simulink model "MSDR_v1.1"  (R2018a)
settings: Solver=ode3  StartTime=0.0  StopTime=21600  FixedStep=0.05
values from neighbouring files (symbols this model uses):
  a_f = -3.22E-5    (= -3.22e-05)    [MSDR_parameters.m]
  a_g = +2.35E-5    (= 2.35e-05)    [MSDR_parameters.m]
  A_s = 1.2245    [MSDR_parameters.m]
  beta = [0.000223, 0.001457, 0.001307, 0.002628, 0.000766, 0.000280]    [MSDR_parameters.m]
  beta_t = sum(beta)    [MSDR_parameters.m]
  ce1 = 1.2471e-07    [MSDR_parameters.m]
  ce2 = 5.3816e-14    [MSDR_parameters.m]
  ce3 = 3.3721e-08    [MSDR_parameters.m]
  Cp_fw = 3200.448e-6    (= 0.003200448)    [MSDR_parameters.m]
  Cp_hr = 0.0021520    (= 0.002152)    [MSDR_parameters.m]
  Cp_p = Cp_s_shx    (= 0.00154912)    [MSDR_parameters.m]
  Cp_s = Cp_s*1e-6    (= 3.588208e-09)    [MSDR_parameters.m]
  Cp_s_shx = 1549.12e-6    (= 0.00154912)    [MSDR_parameters.m]
  Cp_sc = 4761.392e-6    (= 0.004761392)    [MSDR_parameters.m]
  Cp_w = 456.056e-6    (= 0.000456056)    [MSDR_parameters.m]
  D_it = 0.0141478    [MSDR_parameters.m]
  D_ot = 0.015875    [MSDR_parameters.m]
  dHs_dPs = -0.042433622114357    (= -0.0424336221144)    [MSDR_parameters.m]
  eta_hp_isen = 0.861    [MSDR_parameters.m]
  eta_lp_isen = 0.861    [MSDR_parameters.m]
  gamma_I = 5.1135e-2    (= 0.051135)    [MSDR_parameters.m]
  gamma_Xe = 1.1628e-2    (= 0.011628)    [MSDR_parameters.m]
  H_fwh1 = 0.46009    [MSDR_parameters.m]
  h_fwh1 = 0.5927    [MSDR_parameters.m]
  H_fwh2 = 0.6784    [MSDR_parameters.m]
  h_fwh2 = 0.5927    [MSDR_parameters.m]
  H_lp_isen = 958.4*1054.35e-6/0.45359237    (= 2.22774699671)    [MSDR_parameters.m]
  H_nc = 3.2952    [MSDR_parameters.m]
  h_pw = h_s_shx    (= 0.00567446)    [MSDR_parameters.m]
  H_rh = 2.8115    [MSDR_parameters.m]
  h_wb = 13349.334646671E-6    (= 0.0133493346467)    [MSDR_parameters.m]
  h_ws = 5732.378387768E-6    (= 0.00573237838777)    [MSDR_parameters.m]
  h_wsc = 8385.005556375E-6    (= 0.00838500555638)    [MSDR_parameters.m]
  hA_fg = [h_fg*A_fg/2, h_fg*A_fg/2]    [MSDR_parameters.m]
  hA_p_phx1 = h_p_phx*A_p_phx    [MSDR_parameters.m]
  hA_p_phx2 = h_p_phx*A_p_phx    [MSDR_parameters.m]
  hA_p_phx3 = h_p_phx*A_p_phx    [MSDR_parameters.m]
  hA_p_phx4 = h_p_phx*A_p_phx    [MSDR_parameters.m]
  hA_p_phx5 = h_p_phx*A_p_phx    [MSDR_parameters.m]
  hA_p_phx6 = h_p_phx*A_p_phx    [MSDR_parameters.m]
  hA_p_shx1 = h_p_shx*A_p_shx    [MSDR_parameters.m]
  hA_p_shx2 = h_p_shx*A_p_shx    [MSDR_parameters.m]
  hA_p_shx3 = h_p_shx*A_p_shx    [MSDR_parameters.m]
  hA_p_shx4 = h_p_shx*A_p_shx    [MSDR_parameters.m]
  hA_p_shx5 = h_p_shx*A_p_shx    [MSDR_parameters.m]
  hA_p_shx6 = h_p_shx*A_p_shx    [MSDR_parameters.m]
  hA_s_phx1 = h_s_phx*A_s_phx    [MSDR_parameters.m]
  hA_s_phx2 = h_s_phx*A_s_phx    [MSDR_parameters.m]
  hA_s_phx3 = h_s_phx*A_s_phx    [MSDR_parameters.m]
  hA_s_phx4 = h_s_phx*A_s_phx    [MSDR_parameters.m]
  hA_s_phx5 = h_s_phx*A_s_phx    [MSDR_parameters.m]
  hA_s_phx6 = h_s_phx*A_s_phx    [MSDR_parameters.m]
  hA_s_shx1 = h_s_shx*A_s_shx    [MSDR_parameters.m]
  hA_s_shx2 = h_s_shx*A_s_shx    [MSDR_parameters.m]
  hA_s_shx3 = h_s_shx*A_s_shx    [MSDR_parameters.m]
  hA_s_shx4 = h_s_shx*A_s_shx    [MSDR_parameters.m]
  hA_s_shx5 = h_s_shx*A_s_shx    [MSDR_parameters.m]
  hA_s_shx6 = h_s_shx*A_s_shx    [MSDR_parameters.m]
  I_0 = gamma_I*Sig_f_msdr*phi_0/lam_I    (= 4.38204721773e+16)    [MSDR_parameters.m]
  Ifa = [0.25, 0.25]    [MSDR_parameters.m]
  Ifb = [0.25, 0.25]    [MSDR_parameters.m]
  Ig = [0.5, 0.5]    [MSDR_parameters.m]
  K_1 = 11.632248097704855    (= 11.6322480977)    [MSDR_parameters.m]
  K_4 = b(1)    [MSDR_parameters.m]
  K_5 = a(1)    [MSDR_parameters.m]
  K_b = 12.834854076292217    (= 12.8348540763)    [MSDR_parameters.m]
  K_b_hp = 0.1634    [MSDR_parameters.m]
  K_b_lp = 0.2174    [MSDR_parameters.m]
  K_sc = -17.615718797133468    (= -17.6157187971)    [MSDR_parameters.m]
  ka = [0.235, 0.235]    [MSDR_parameters.m]
  kb = [0.235, 0.235]    [MSDR_parameters.m]
  kga = [0.015, 0.015]    [MSDR_parameters.m]
  kgb = [0.015, 0.015]    [MSDR_parameters.m]
  L = 8.5344    [MSDR_parameters.m]
  L_b = 2.3645    [MSDR_parameters.m]
  L_s = 4.723    [MSDR_parameters.m]
  Lam = 2.400E-04    (= 0.00024)    [MSDR_parameters.m]
  lam = [0.0124, 0.0305, 0.111, 0.301, 1.14, 3.01]    [MSDR_parameters.m]
  lam_bubl = 2.0e-2    (= 0.02)    [MSDR_parameters.m]
  lam_I = 2.875e-5    (= 2.875e-05)    [MSDR_parameters.m]
  lam_Xe = 2.0916e-5    (= 2.0916e-05)    [MSDR_parameters.m]
  m_3m = W_3*2    (= 8618.207327)    [MSDR_parameters.m]
  m_fm = W_f*2    (= 9978.96)    [MSDR_parameters.m]
  m_sb = 1717    [MSDR_parameters.m]
  M_stm = 0.018    [MSDR_parameters.m]
  mb_cpb = 2.689619410657651e+00    (= 2.68961941066)    [MSDR_parameters.m]
  mcp_fa = mfa*Cp_f    [MSDR_parameters.m]
  mcp_fb = mfb*Cp_f    [MSDR_parameters.m]
  mcp_g = mg*Cp_g    [MSDR_parameters.m]
  mcp_p_phx1 = Cp_p_phx*mp_phx1    [MSDR_parameters.m]
  mcp_p_phx2 = Cp_p_phx*mp_phx2    [MSDR_parameters.m]
  mcp_p_phx3 = Cp_p_phx*mp_phx3    [MSDR_parameters.m]
  mcp_p_phx4 = Cp_p_phx*mp_phx4    [MSDR_parameters.m]
  mcp_p_phx5 = Cp_p_phx*mp_phx5    [MSDR_parameters.m]
  mcp_p_phx6 = Cp_p_phx*mp_phx6    [MSDR_parameters.m]
  mcp_p_shx1 = Cp_p_shx*mp_shx1    [MSDR_parameters.m]
  mcp_p_shx2 = Cp_p_shx*mp_shx2    [MSDR_parameters.m]
  mcp_p_shx3 = Cp_p_shx*mp_shx3    [MSDR_parameters.m]
  mcp_p_shx4 = Cp_p_shx*mp_shx4    [MSDR_parameters.m]
  mcp_p_shx5 = Cp_p_shx*mp_shx5    [MSDR_parameters.m]
  mcp_p_shx6 = Cp_p_shx*mp_shx6    [MSDR_parameters.m]
  mcp_s_phx1 = Cp_s_phx*ms_phx1    [MSDR_parameters.m]
  mcp_s_phx2 = Cp_s_phx*ms_phx2    [MSDR_parameters.m]
  mcp_s_phx3 = Cp_s_phx*ms_phx3    [MSDR_parameters.m]
  mcp_s_phx4 = Cp_s_phx*ms_phx4    [MSDR_parameters.m]
  mcp_s_phx5 = Cp_s_phx*ms_phx5    [MSDR_parameters.m]
  mcp_s_phx6 = Cp_s_phx*ms_phx6    [MSDR_parameters.m]
  mcp_s_shx1 = Cp_s_shx*ms_shx1    [MSDR_parameters.m]
  mcp_s_shx2 = Cp_s_shx*ms_shx1    [MSDR_parameters.m]
  mcp_s_shx3 = Cp_s_shx*ms_shx1    [MSDR_parameters.m]
  mcp_s_shx4 = Cp_s_shx*ms_shx1    [MSDR_parameters.m]
  mcp_s_shx5 = Cp_s_shx*ms_shx1    [MSDR_parameters.m]
  mcp_s_shx6 = Cp_s_shx*ms_shx1    [MSDR_parameters.m]
  mcp_t_phx1 = Cp_t_phx*mt_phx1    [MSDR_parameters.m]
  mcp_t_phx2 = Cp_t_phx*mt_phx2    [MSDR_parameters.m]
  mcp_t_phx3 = Cp_t_phx*mt_phx3    [MSDR_parameters.m]
  mcp_t_phx4 = Cp_t_phx*mt_phx4    [MSDR_parameters.m]
  mcp_t_phx5 = Cp_t_phx*mt_phx5    [MSDR_parameters.m]
  mcp_t_phx6 = Cp_t_phx*mt_phx6    [MSDR_parameters.m]
  mcp_t_shx1 = Cp_t_phx*mt_shx1    [MSDR_parameters.m]
  ... (+177 more)
undefined symbols (not defined in the file or in its folder): C0, H_rh_table, H_rh_table1, H_rh_table2, H_rhvap_table, H_s_table, H_table, hA_p_thx1, hA_p_thx2, hA_p_thx3, hA_s_thx1, hA_s_thx2, hA_s_thx3, mcp_p_thx1, mcp_p_thx2, mcp_p_thx3, mcp_s_thx1, mcp_s_thx2, mcp_s_thx3, mcp_t_thx1, mcp_t_thx2, mcp_t_thx3, mp_thx1, mp_thx2, mp_thx3, ms_thx1, ms_thx2, ms_thx3, P_nc_table, P_rh_table, P_rh_table1, pres_table, rho_rh_table, rho_table, SV_nc_table, T0_p_thx1, T0_p_thx2, T0_p_thx3, T0_s_thx1, T0_s_thx2, T0_s_thx3, T0_t_thx1, T0_t_thx2, T0_t_thx3, temp_table, u14, Wp_thx1, Wp_thx2
libraries: simulink x13
(part 1 of 6)
settings Model: Creator=viikr  LastModifiedBy=Vikram Singh
settings SolverCC: AlgebraicLoopSolver=LineSearch

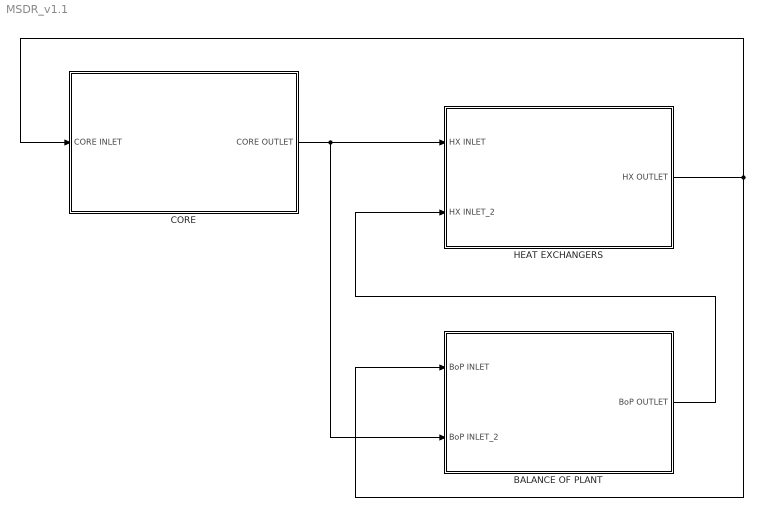
== system MSDR_v1.1 ==
  BALANCE OF PLANT : Subsystem
  CORE : Subsystem
  HEAT EXCHANGERS : Subsystem
  wires:
  BALANCE OF PLANT/1(BoP OUTLET) -> HEAT EXCHANGERS/2(HX INLET_2)
  HEAT EXCHANGERS/1(HX OUTLET) -> BALANCE OF PLANT/1(BoP INLET), CORE/1(CORE INLET)
  CORE/1(CORE OUTLET) -> BALANCE OF PLANT/2(BoP INLET_2), HEAT EXCHANGERS/1(HX INLET)

== system MSDR_v1.1/BALANCE OF PLANT ==
  In Bus Element : Inport  PortName=BoP INLET  Element=HX HITEC OUTLET TEMPERATURE
  In Bus Element1 : Inport  Port=2  PortName=BoP INLET_2  Element=CORE POWER
  Constant : Constant  Value=425
  POWER : Subsystem
  Bus Element Out2 : Outport  PortName=BoP OUTLET  Element=BoP HITEC OUTLET TEMPERATURE
  wires:
  In Bus Element/1 -> POWER/1(HITEC_INLET)
  In Bus Element1/1 -> POWER/2(POWER LEVEL)
  POWER/1(HITEC_OUTLET) -> Bus Element Out2/1

== system MSDR_v1.1/CORE ==
  In Bus Element2 : Inport  PortName=CORE INLET  Element=FUEL HEAT TRANSFER FRACTION
  In Bus Element : Inport  PortName=CORE INLET  Element=HX FUEL OUTLET TEMPERATURE
  In Bus Element1 : Inport  PortName=CORE INLET  Element=FUEL FLOW FRACTION
  CORE HEAT TRANSFER : Subsystem
  CORE TO HX DELAY : VariableTransportDelay  MaximumDelay=10000000  InitialOutput=T0_fb(2)
  PKE SOLVER : Subsystem
  REACTIVITY : Subsystem
  REACTIVITY1 : Subsystem
  Tf_out : Fcn  Expr=u[7]
  VAR DELAY FUNC : Fcn  Expr=tau_c_hx/u
  Bus Element Out2 : Outport  PortName=CORE OUTLET  Element=CORE FUEL OUTLET TEMPERATURE
  Bus Element Out1 : Outport  PortName=CORE OUTLET  Element=CORE POWER
  wires:
  Tf_out/1 -> CORE TO HX DELAY/1
  CORE HEAT TRANSFER/1(CORE TEMPERATURES) -> [Tf_out], Tf_out/1
  [Tf_out] -> REACTIVITY/1(CORE TEMPERATURES)
  PKE SOLVER/1(FRACTIONAL NEUTRON DENSITY) -> Bus Element Out1/1, [Frac_neut]
  [Frac_neut] -> CORE HEAT TRANSFER/1(FRACTIONAL NEUTRON DENSITY)
  REACTIVITY/1(TOTAL REACTIVITY FEEDBACK) -> [rho_tot]
  [flow_frac] -> PKE SOLVER/2(FLOW FRACTION)
  [flow_frac] -> CORE HEAT TRANSFER/3(FLOW FRACTION)
  [hA_frac] -> CORE HEAT TRANSFER/4(HEAT TRANSFER FRACTION)
  CORE TO HX DELAY/1 -> Bus Element Out2/1
  [flow_frac] -> VAR DELAY FUNC/1
  VAR DELAY FUNC/1 -> CORE TO HX DELAY/2
  [Tf_in] -> CORE HEAT TRANSFER/2(FUEL INLET TEMPERATURE)
  REACTIVITY1/1(drho_Xe) -> [drho_Xe]
  [Frac_neut] -> REACTIVITY1/1(n0)
  In Bus Element1/1 -> [flow_frac]
  In Bus Element2/1 -> [hA_frac]
  In Bus Element/1 -> [Tf_in]
  [drho_Xe] -> REACTIVITY/2(XENON REACTIVITY)
  [rho_tot] -> PKE SOLVER/1(REACTIVITY FEEDBACK)

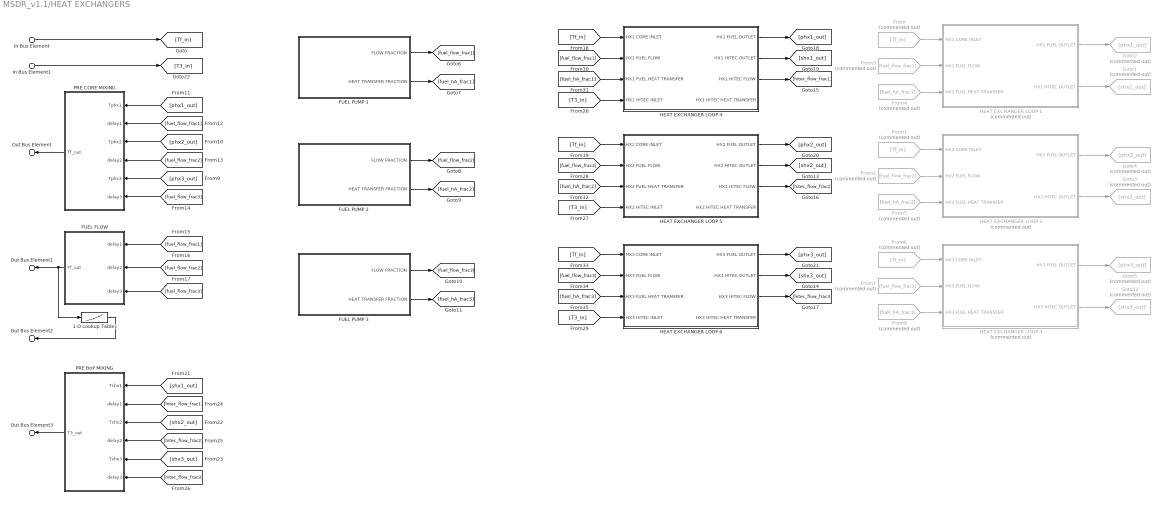
== system MSDR_v1.1/HEAT EXCHANGERS ==
  In Bus Element : Inport  PortName=HX INLET  Element=CORE FUEL OUTLET TEMPERATURE
  In Bus Element1 : Inport  Port=2  PortName=HX INLET_2  Element=BoP HITEC OUTLET TEMPERATURE
  1-D Lookup Table1 : Lookup_n-D  NumberOfTableDimensions=1  BreakpointsForDimension1=xdat  Table=ydat  InternalRulePriority=Speed  RndMeth=Simplest  InputSameDT=on
  FUEL FLOW : Subsystem
  FUEL PUMP 1 : Subsystem
  FUEL PUMP 2 : Subsystem
  FUEL PUMP 3 : Subsystem
  From : From  Commented=on  GotoTag=Tf_in
  From1 : From  Commented=on  GotoTag=Tf_in
  From2 : From  Commented=on  GotoTag=fuel_flow_frac2
  From3 : From  Commented=on  GotoTag=fuel_flow_frac1
  From4 : From  Commented=on  GotoTag=fuel_hA_frac1
  From5 : From  Commented=on  GotoTag=fuel_hA_frac2
  From6 : From  Commented=on  GotoTag=Tf_in
  From7 : From  Commented=on  GotoTag=fuel_flow_frac3
  From8 : From  Commented=on  GotoTag=fuel_hA_frac3
  Goto1 : Goto  Commented=on  GotoTag=shx1_out
  Goto12 : Goto  Commented=on  GotoTag=shx3_out
  Goto2 : Goto  Commented=on  GotoTag=phx1_out
  Goto3 : Goto  Commented=on  GotoTag=shx2_out
  Goto4 : Goto  Commented=on  GotoTag=phx2_out
  Goto5 : Goto  Commented=on  GotoTag=phx3_out
  HEAT EXCHANGER LOOP 1 : Subsystem  Commented=on
  HEAT EXCHANGER LOOP 2 : Subsystem  Commented=on
  HEAT EXCHANGER LOOP 3 : Subsystem  Commented=on
  HEAT EXCHANGER LOOP 4 : Subsystem
  HEAT EXCHANGER LOOP 5 : Subsystem
  HEAT EXCHANGER LOOP 6 : Subsystem
  PRE BoP MIXING : Subsystem
  PRE CORE MIXING : Subsystem
  Out Bus Element : Outport  PortName=HX OUTLET  Element=HX FUEL OUTLET TEMPERATURE
  Out Bus Element1 : Outport  PortName=HX OUTLET  Element=FUEL FLOW FRACTION
  Out Bus Element2 : Outport  PortName=HX OUTLET  Element=FUEL HEAT TRANSFER FRACTION
  Out Bus Element3 : Outport  PortName=HX OUTLET  Element=HX HITEC OUTLET TEMPERATURE
  wires:
  From/1 -> HEAT EXCHANGER LOOP 1/1(HX1 CORE INLET)
  From3/1 -> HEAT EXCHANGER LOOP 1/2(HX1 FUEL FLOW)
  From4/1 -> HEAT EXCHANGER LOOP 1/3(HX1 FUEL HEAT TRANSFER)
  From1/1 -> HEAT EXCHANGER LOOP 2/1(HX2 CORE INLET)
  From5/1 -> HEAT EXCHANGER LOOP 2/3(HX2 FUEL HEAT TRANSFER)
  From2/1 -> HEAT EXCHANGER LOOP 2/2(HX2 FUEL FLOW)
  From6/1 -> HEAT EXCHANGER LOOP 3/1(HX3 CORE INLET)
  From7/1 -> HEAT EXCHANGER LOOP 3/2(HX3 FUEL FLOW)
  From8/1 -> HEAT EXCHANGER LOOP 3/3(HX3 FUEL HEAT TRANSFER)
  In Bus Element/1 -> [Tf_in]
  HEAT EXCHANGER LOOP 1/1(HX1 FUEL OUTLET) -> Goto2/1
  HEAT EXCHANGER LOOP 2/1(HX2 FUEL OUTLET) -> Goto4/1
  HEAT EXCHANGER LOOP 3/1(HX3 FUEL OUTLET) -> Goto5/1
  FUEL PUMP 1/1(FLOW FRACTION) -> [fuel_flow_frac1]
  FUEL PUMP 1/2(HEAT TRANSFER FRACTION) -> [fuel_hA_frac1]
  FUEL PUMP 2/2(HEAT TRANSFER FRACTION) -> [fuel_hA_frac2]
  FUEL PUMP 2/1(FLOW FRACTION) -> [fuel_flow_frac2]
  FUEL PUMP 3/2(HEAT TRANSFER FRACTION) -> [fuel_hA_frac3]
  FUEL PUMP 3/1(FLOW FRACTION) -> [fuel_flow_frac3]
  [phx1_out] -> PRE CORE MIXING/1(Tphx1)
  [fuel_flow_frac1] -> PRE CORE MIXING/2(delay1)
  [phx2_out] -> PRE CORE MIXING/3(Tphx2)
  [fuel_flow_frac2] -> PRE CORE MIXING/4(delay2)
  [phx3_out] -> PRE CORE MIXING/5(Tphx3)
  [fuel_flow_frac3] -> PRE CORE MIXING/6(delay3)
  PRE CORE MIXING/1(Tf_out) -> Out Bus Element/1
  [fuel_flow_frac2] -> FUEL FLOW/2(delay2)
  [fuel_flow_frac1] -> FUEL FLOW/1(delay1)
  [fuel_flow_frac3] -> FUEL FLOW/3(delay3)
  FUEL FLOW/1(Tf_out) -> 1-D Lookup Table1/1, Out Bus Element1/1
  1-D Lookup Table1/1 -> Out Bus Element2/1
  [hitec_flow_frac2] -> PRE BoP MIXING/4(delay2)
  [hitec_flow_frac1] -> PRE BoP MIXING/2(delay1)
  [shx2_out] -> PRE BoP MIXING/3(Tshx2)
  [shx3_out] -> PRE BoP MIXING/5(Tshx3)
  [hitec_flow_frac3] -> PRE BoP MIXING/6(delay3)
  [shx1_out] -> PRE BoP MIXING/1(Tshx1)
  PRE BoP MIXING/1(T3_out) -> Out Bus Element3/1
  HEAT EXCHANGER LOOP 1/2(HX1 HITEC OUTLET) -> Goto1/1
  HEAT EXCHANGER LOOP 2/2(HX2 HITEC OUTLET) -> Goto3/1
  HEAT EXCHANGER LOOP 3/2(HX3 HITEC OUTLET) -> Goto12/1
  HEAT EXCHANGER LOOP 5/2(HX2 HITEC OUTLET) -> [shx2_out]
  [T3_in] -> HEAT EXCHANGER LOOP 6/4(HX3 HITEC INLET)
  HEAT EXCHANGER LOOP 6/3(HX3 HITEC FLOW) -> [hitec_flow_frac3]
  HEAT EXCHANGER LOOP 5/3(HX2 HITEC FLOW) -> [hitec_flow_frac2]
  HEAT EXCHANGER LOOP 4/3(HX1 HITEC FLOW) -> [hitec_flow_frac1]
  HEAT EXCHANGER LOOP 6/2(HX3 HITEC OUTLET) -> [shx3_out]
  HEAT EXCHANGER LOOP 4/2(HX1 HITEC OUTLET) -> [shx1_out]
  [T3_in] -> HEAT EXCHANGER LOOP 4/4(HX1 HITEC INLET)
  HEAT EXCHANGER LOOP 4/1(HX1 FUEL OUTLET) -> [phx1_out]
  [fuel_flow_frac3] -> HEAT EXCHANGER LOOP 6/2(HX3 FUEL FLOW)
  [Tf_in] -> HEAT EXCHANGER LOOP 5/1(HX2 CORE INLET)
  [T3_in] -> HEAT EXCHANGER LOOP 5/4(HX2 HITEC INLET)
  [fuel_hA_frac2] -> HEAT EXCHANGER LOOP 5/3(HX2 FUEL HEAT TRANSFER)
  [fuel_flow_frac1] -> HEAT EXCHANGER LOOP 4/2(HX1 FUEL FLOW)
  [fuel_flow_frac2] -> HEAT EXCHANGER LOOP 5/2(HX2 FUEL FLOW)
  [Tf_in] -> HEAT EXCHANGER LOOP 6/1(HX3 CORE INLET)
  [fuel_hA_frac1] -> HEAT EXCHANGER LOOP 4/3(HX1 FUEL HEAT TRANSFER)
  [Tf_in] -> HEAT EXCHANGER LOOP 4/1(HX1 CORE INLET)
  [fuel_hA_frac3] -> HEAT EXCHANGER LOOP 6/3(HX3 FUEL HEAT TRANSFER)
  HEAT EXCHANGER LOOP 6/1(HX3 FUEL OUTLET) -> [phx3_out]
  HEAT EXCHANGER LOOP 5/1(HX2 FUEL OUTLET) -> [phx2_out]
  In Bus Element1/1 -> [T3_in]

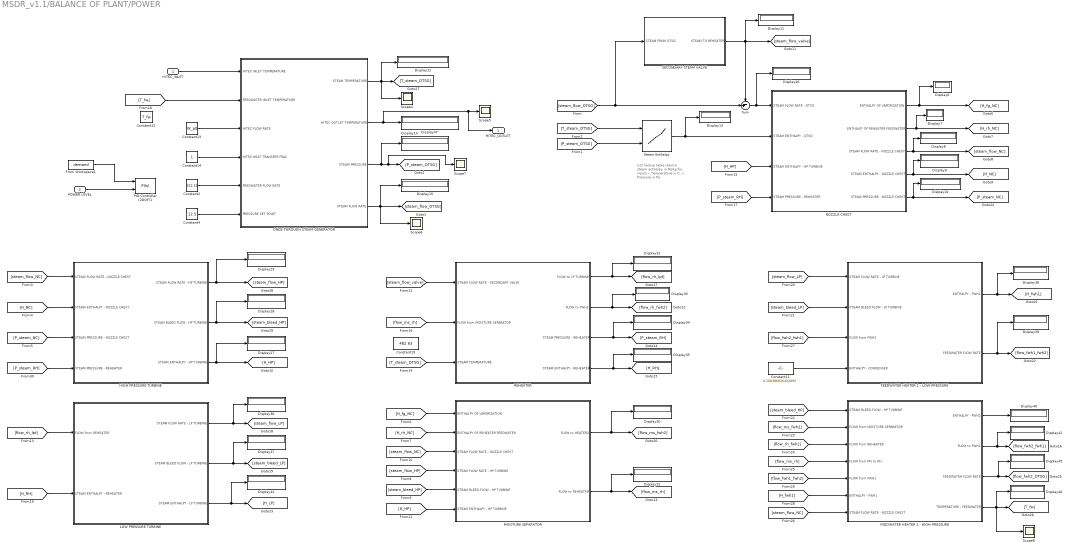
== system MSDR_v1.1/BALANCE OF PLANT/POWER ==
  note: 2-D lookup table returns steam enthalpy in MJ/kg for inputs i. Temperature in C, ii. Pressure in Pa
  HITEC_INLET : Inport
  POWER LEVEL : Inport  Port=2
  Constant11 : Constant  Value=0.160386626432892
  Constant12 : Constant  Value=T_fw
  Constant13 : Constant  Value=W_p0
  Constant14 : Constant
  Constant19 : Constant  Value=482.63
  Constant2 : Constant  Value=322.22
  Constant4 : Constant  Value=12.5
  Display{6..15,26..42,45..47} (30 alike) : Display
  FEEDWATER HEATER 1 - LOW-PRESSURE : Subsystem
  FEEDWATER HEATER 2 - HIGH-PRESSURE : Subsystem
  From Workspace1 : FromWorkspace  VariableName=demand  SampleTime=1  Interpolate=off  OutputAfterFinalValue=Holding final value
  HIGH PRESSURE TURBINE : Subsystem
  LOW PRESSURE TURBINE : Subsystem
  MOISTURE SEPARATOR : Subsystem
  NOZZLE CHEST : Subsystem
  ONCE-THROUGH STEAM GENERATOR : Subsystem
  PID Controller (2DOF)1 : simulink/Continuous/PID Controller (2DOF)  Controller=PI  TimeDomain=Continuous-time  SampleTime=-1  IntegratorMethod=Forward Euler  FilterMethod=Forward Euler  Form=Parallel  UseFilter=on  ControllerParametersSource=internal  P=250  I=5  D=1  N=100  b=1  c=1  InitialConditionSource=internal  InitialConditionForIntegrator=0  InitialConditionForFilter=0  ExternalReset=none  LimitOutput=on  UpperSaturationLimit=1000  LowerSaturationLimit=100  LinearizeAsGain=on  AntiWindupMode=none  Kb=1  TrackingMode=off  Kt=1  PParamMin=[]  PParamMax=[]  IParamMin=[]  IParamMax=[]  DParamMin=[]  DParamMax=[]  NParamMin=[]  NParamMax=[]  bParamMin=[]  bParamMax=[]  cParamMin=[]  cParamMax=[]  KbParamMin=[]  KbParamMax=[]  KtParamMin=[]  KtParamMax=[]  POutMin=[]  POutMax=[]  IOutMin=[]  IOutMax=[]  DOutMin=[]  DOutMax=[]  NOutMin=[]  NOutMax=[]  bOutMin=[]  bOutMax=[]  cOutMin=[]  cOutMax=[]  KbOutMin=[]  KbOutMax=[]  KtOutMin=[]  KtOutMax=[]  IntegratorOutMin=[]  IntegratorOutMax=[]  FilterOutMin=[]  FilterOutMax=[]  SumOutMin=[]  SumOutMax=[]  Sum1OutMin=[]  Sum1OutMax=[]  Sum2OutMin=[]  Sum2OutMax=[]  Sum3OutMin=[]  Sum3OutMax=[]  SumI1OutMin=[]  SumI1OutMax=[]  SumI2OutMin=[]  SumI2OutMax=[]  SumI3OutMin=[]  SumI3OutMax=[]  SumDOutMin=[]  SumDOutMax=[]  SaturationOutMin=[]  SaturationOutMax=[]  IntegratorContinuousStateAttributes=''  IntegratorStateMustResolveToSignalObject=off  IntegratorRTWStateStorageClass=Auto  FilterContinuousStateAttributes=''  FilterStateMustResolveToSignalObject=off  FilterRTWStateStorageClass=Auto  DifferentiatorICPrevScaledInput=0  DifferentiatorOutMin=[]  DifferentiatorOutMax=[]  FilterDiffOutCoefMin=[]  FilterDiffOutCoefMax=[]  SumDenOutMin=[]  SumDenOutMax=[]  SumNumOutMin=[]  SumNumOutMax=[]  ReciprocalOutMin=[]  ReciprocalOutMax=[]  DivideOutMin=[]  DivideOutMax=[]  TunerSelectOption=Transfer Function Based (PID Tuner App)
  REHEATER : Subsystem
  SECONDARY STEAM VALVE : Subsystem
  Scope{4..8} (5 alike) : Scope
  Steam Enthalpy : Lookup_n-D  BreakpointsForDimension1=temp_table  BreakpointsForDimension2=pres_table  Table=H_s_table  DiagnosticForOutOfRangeInput=Warning  InternalRulePriority=Speed  RndMeth=Simplest  InputSameDT=on
  Sum : Sum  Inputs=-+|
  HITEC_OUTLET : Outport
  wires:
  REHEATER/1("FLOW to LP TURBINE ") -> [flow_rh_lpt], Display32/1
  [steam_flow_NC] -> HIGH PRESSURE TURBINE/1(STEAM FLOW RATE - NOZZLE CHEST)
  [steam_bleed_HP] -> MOISTURE SEPARATOR/5(STEAM BLEED FLOW - HP TURBINE)
  [steam_flow_NC] -> MOISTURE SEPARATOR/3(STEAM FLOW RATE - NOZZLE CHEST)
  NOZZLE CHEST/3(STEAM FLOW RATE - NOZZLE CHEST) -> [steam_flow_NC], Display8/1
  [H_rh_NC] -> MOISTURE SEPARATOR/2(ENTHALPY OF REHEATER FEEDWATER)
  NOZZLE CHEST/2(ENTHALPY OF REHEATER FEEDWATER) -> [H_rh_NC], Display7/1
  [H_NC] -> HIGH PRESSURE TURBINE/2(STEAM ENTHALPY - NOZZLE CHEST)
  Steam Enthalpy/1 -> NOZZLE CHEST/2(STEAM ENTHALPY - OTSG), Display13/1
  [steam_flow_HP] -> MOISTURE SEPARATOR/4(STEAM FLOW RATE - HP TURBINE)
  Sum/1 -> Display26/1, NOZZLE CHEST/1(STEAM FLOW RATE - OTSG)
  NOZZLE CHEST/5(STEAM PRESSURE - NOZZLE CHEST) -> [P_steam_NC], Display10/1
  [H_fwh1] -> FEEDWATER HEATER 2 - HIGH-PRESSURE/6(ENTHALPY - FWH1)
  REHEATER/2(FLOW to FWH2) -> [flow_rh_fwh2], Display33/1
  FEEDWATER HEATER 1 - LOW-PRESSURE/1(ENTHALPY - FWH1) -> [H_fwh1], Display38/1
  [flow_rh_fwh2] -> FEEDWATER HEATER 2 - HIGH-PRESSURE/3(FLOW from REHEATER)
  [flow_ms_rh] -> FEEDWATER HEATER 2 - HIGH-PRESSURE/4(FLOW from MS to RH)
  FEEDWATER HEATER 2 - HIGH-PRESSURE/2(FLOW to FWH1) -> Display41/1, [flow_fwh2_fwh1]
  [flow_ms_fwh2] -> FEEDWATER HEATER 2 - HIGH-PRESSURE/2(FLOW from MOISTURE SEPARATOR)
  [steam_flow_LP] -> FEEDWATER HEATER 1 - LOW-PRESSURE/1(STEAM FLOW RATE - LP TURBINE)
  MOISTURE SEPARATOR/1(FLOW to HEATER2) -> [flow_ms_fwh2], Display30/1
  [flow_fwh2_fwh1] -> FEEDWATER HEATER 1 - LOW-PRESSURE/3(FLOW from FWH2)
  [flow_ms_rh] -> REHEATER/2(FLOW from MOISTURE SEPARATOR)
  MOISTURE SEPARATOR/2(FLOW to REHEATER) -> [flow_ms_rh], Display31/1
  REHEATER/3(STEAM PRESSURE - REHEATER) -> [P_steam_RH], Display34/1
  FEEDWATER HEATER 2 - HIGH-PRESSURE/3(FEEDWATER FLOW RATE) -> Display45/1, [flow_fwh2_OTSG]
  LOW PRESSURE TURBINE/3(STEAM ENTHALPY - LP TURBINE) -> Display42/1, [H_LP]
  [P_steam_NC] -> HIGH PRESSURE TURBINE/3(STEAM PRESSURE - NOZZLE CHEST)
  FEEDWATER HEATER 2 - HIGH-PRESSURE/4(TEMPERATURE - FEEDWATER) -> [T_fw], Scope8/1, Display46/1
  NOZZLE CHEST/4(STEAM ENTHALPY - NOZZLE CHEST) -> [H_NC], Display9/1
  [flow_rh_lpt] -> LOW PRESSURE TURBINE/1(FLOW from REHEATER)
  HIGH PRESSURE TURBINE/3(STEAM ENTHALPY - HP TURBINE) -> [H_HP], Display27/1
  [H_fg_NC] -> MOISTURE SEPARATOR/1(ENTHALPY OF VAPORIZATION)
  [flow_fwh1_fwh2] -> FEEDWATER HEATER 2 - HIGH-PRESSURE/5(FLOW from FWH1)
  [steam_flow_valve] -> REHEATER/1(STEAM FLOW RATE - SECONDARY VALVE)
  ONCE-THROUGH STEAM GENERATOR/4(STEAM FLOW RATE) -> Scope6/1, [steam_flow_OTSG], Display15/1
  [P_steam_OTSG] -> Steam Enthalpy/2
  [H_HP] -> MOISTURE SEPARATOR/6(STEAM ENTHALPY - HP TURBINE)
  SECONDARY STEAM VALVE/1(STEAM TO REHEATER) -> [steam_flow_valve], Display11/1, Sum/1
  [H_HP] -> NOZZLE CHEST/3(STEAM ENTHALPY - HP TURBINE)
  ONCE-THROUGH STEAM GENERATOR/2(HITEC OUTLET TEMPERATURE) -> HITEC_OUTLET/1, Scope5/1, Display47/1
  NOZZLE CHEST/1(ENTHALPY OF VAPORIZATION) -> [H_fg_NC], Display6/1
  [P_steam_RH] -> NOZZLE CHEST/4(STEAM PRESSURE - REHEATER)
  REHEATER/4(STEAM ENTHALPY - REHEATER) -> [H_RH], Display35/1
  LOW PRESSURE TURBINE/2(STEAM BLEED FLOW - LP TURBINE) -> [steam_bleed_LP], Display37/1
  Constant13/1 -> ONCE-THROUGH STEAM GENERATOR/3(HITEC FLOW RATE)
  Constant11/1 -> FEEDWATER HEATER 1 - LOW-PRESSURE/4(ENTHALPY - CONDENSER)
  FEEDWATER HEATER 2 - HIGH-PRESSURE/1(ENTHALPY - FWH2) -> Display40/1
  HIGH PRESSURE TURBINE/1(STEAM FLOW RATE - HP TURBINE) -> [steam_flow_HP], Display29/1
  [T_steam_OTSG] -> REHEATER/3(STEAM TEMPERATURE)
  ONCE-THROUGH STEAM GENERATOR/1(STEAM TEMPERATURE) -> Scope4/1, Display12/1, [T_steam_OTSG]
  Constant14/1 -> ONCE-THROUGH STEAM GENERATOR/4(HITEC HEAT TRANSFER FRAC)
  [T_fw] -> ONCE-THROUGH STEAM GENERATOR/2(FEEDWATER INLET TEMPERATURE)
  [steam_bleed_LP] -> FEEDWATER HEATER 1 - LOW-PRESSURE/2(STEAM BLEED FLOW - LP TURBINE)
  [H_RH] -> LOW PRESSURE TURBINE/2(STEAM ENTHALPY - REHEATER)
  Constant4/1 -> ONCE-THROUGH STEAM GENERATOR/6(PRESSURE SET POINT)
  [steam_bleed_HP] -> FEEDWATER HEATER 2 - HIGH-PRESSURE/1(STEAM BLEED FLOW - HP TURBINE)
  ONCE-THROUGH STEAM GENERATOR/3(STEAM PRESSURE) -> Scope7/1, [P_steam_OTSG], Display14/1
  LOW PRESSURE TURBINE/1(STEAM FLOW RATE - LP TURBINE) -> [steam_flow_LP], Display36/1
  [T_steam_OTSG] -> Steam Enthalpy/1
  [P_steam_RH] -> HIGH PRESSURE TURBINE/4(STEAM PRESSURE - REHEATER)
  HIGH PRESSURE TURBINE/2(STEAM BLEED FLOW - HP TURBINE) -> [steam_bleed_HP], Display28/1
  [steam_flow_NC] -> FEEDWATER HEATER 2 - HIGH-PRESSURE/7(STEAM FLOW RATE - NOZZLE CHEST)
  FEEDWATER HEATER 1 - LOW-PRESSURE/2(FEEDWATER FLOW RATE) -> Display39/1, [flow_fwh1_fwh2]
  [steam_flow_OTSG] -> SECONDARY STEAM VALVE/1(STEAM FROM OTSG), Sum/2
  HITEC_INLET/1 -> ONCE-THROUGH STEAM GENERATOR/1(HITEC INLET TEMPERATURE)
  POWER LEVEL/1 -> PID Controller (2DOF)1/2
  From Workspace1/1 -> PID Controller (2DOF)1/1
  Constant2/1 -> ONCE-THROUGH STEAM GENERATOR/5(FEEDWATER FLOW RATE)

== system MSDR_v1.1/CORE/CORE HEAT TRANSFER ==
  FRACTIONAL NEUTRON DENSITY : Inport
  FUEL INLET TEMPERATURE : Inport  Port=2
  FLOW FRACTION : Inport  Port=3
  HEAT TRANSFER FRACTION : Inport  Port=4
  Mux : Mux  Inputs=10
      settings: DisplayOption=signals
  T_f1a : Integrator  InitialCondition=T0_fa(1)
  T_f1b : Integrator  InitialCondition=T0_fb(1)
  T_f2a : Integrator  InitialCondition=T0_fa(2)
  T_f2b : Integrator  InitialCondition=T0_fb(2)
  T_g1 : Integrator  InitialCondition=T0_g(1)
  T_g2 : Integrator  InitialCondition=T0_g(2)
  To Workspace : ToWorkspace  VariableName=core_ht  SampleTime=-1
  d(T_f1a)/dt : Fcn  Expr=((u[9]*W_f/mfa(1))*(u[2] - u[3])) + (ka(1)*P*u[1]/mcp_fa(1)) + (kga(1)*u[10]*hA_fg(1)*(u[5] - u[3]))/((kga(1)+kgb(1))*mcp_fa(1))
  d(T_f1b)/dt : Fcn  Expr=((u[9]*W_f/mfb(1))*(u[3] - u[4])) + (kb(1)*P*u[1]/mcp_fb(1)) + (kgb(1)*u[10]*hA_fg(1)*(u[5] - u[3]))/((kga(1)+kgb(1))*mcp_fb(1))
  d(T_f2a)/dt : Fcn  Expr=((u[9]*W_f/mfa(2))*(u[4] - u[6])) + (ka(2)*P*u[1]/mcp_fa(2)) + (kga(2)*u[10]*hA_fg(2)*(u[8] - u[6]))/((kga(2)+kgb(2))*mcp_fa(2))
  d(T_f2b)/dt : Fcn  Expr=((u[9]*W_f/mfb(2))*(u[6] - u[7])) + (kb(2)*P*u[1]/mcp_fb(2)) + (kgb(2)*u[10]*hA_fg(2)*(u[8] - u[6]))/((kga(2)+kgb(2))*mcp_fb(2))
  d(T_g1)/dt : Fcn  Expr=(u[10]*hA_fg(1)/mcp_g(1))*(u[3] - u[5]) + (kga(1)+kgb(1))*P*u[1]/mcp_g(1)
  d(T_g2)/dt : Fcn  Expr=(u[10]*hA_fg(2)/mcp_g(2))*(u[6] - u[8]) + (kga(2)+kgb(2))*P*u[1]/mcp_g(2)
  CORE TEMPERATURES : Outport
  wires:
  FRACTIONAL NEUTRON DENSITY/1 -> Mux/1
  d(T_f1b)/dt/1 -> T_f1b/1
  d(T_f1a)/dt/1 -> T_f1a/1
  d(T_g1)/dt/1 -> T_g1/1
  FUEL INLET TEMPERATURE/1 -> Mux/2
  T_f1a/1 -> Mux/3
  T_f1b/1 -> Mux/4
  T_g1/1 -> Mux/5
  d(T_f2a)/dt/1 -> T_f2a/1
  d(T_f2b)/dt/1 -> T_f2b/1
  T_g2/1 -> Mux/8
  d(T_g2)/dt/1 -> T_g2/1
  T_f2a/1 -> Mux/6
  T_f2b/1 -> Mux/7
  Mux/1 -> d(T_g2)/dt/1, d(T_f2b)/dt/1, d(T_f2a)/dt/1, d(T_g1)/dt/1, d(T_f1b)/dt/1, d(T_f1a)/dt/1, CORE TEMPERATURES/1, To Workspace/1
  FLOW FRACTION/1 -> Mux/9
  HEAT TRANSFER FRACTION/1 -> Mux/10

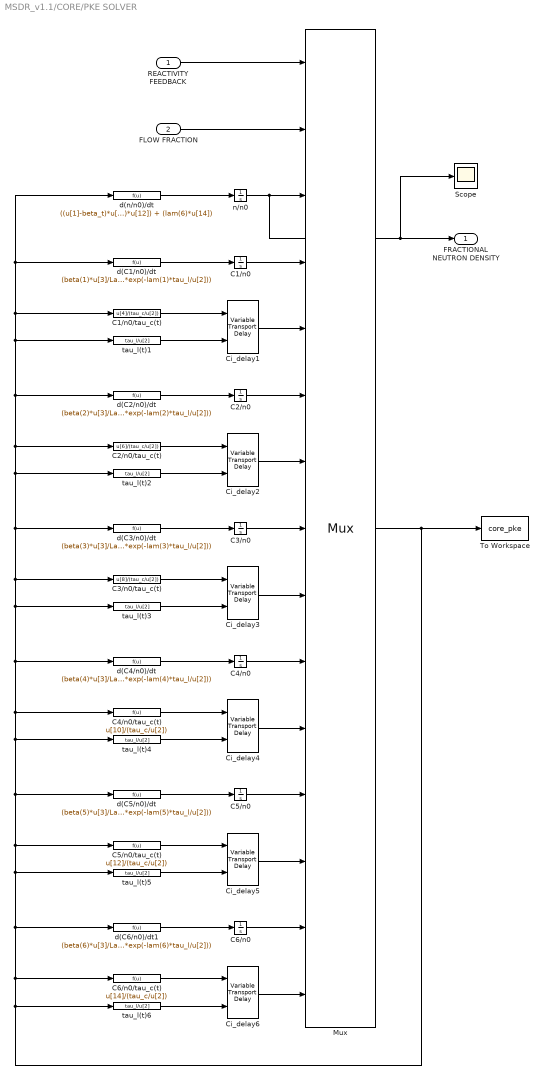
== system MSDR_v1.1/CORE/PKE SOLVER ==
  REACTIVITY FEEDBACK : Inport
  FLOW FRACTION : Inport  Port=2
  C1/n0 : Integrator  InitialCondition=C0(1)
  C1/n0/tau_c(t) : Fcn  Expr=u[4]/(tau_c/u[2])
  C2/n0 : Integrator  InitialCondition=C0(2)
  C2/n0/tau_c(t) : Fcn  Expr=u[6]/(tau_c/u[2])
  C3/n0 : Integrator  InitialCondition=C0(3)
  C3/n0/tau_c(t) : Fcn  Expr=u[8]/(tau_c/u[2])
  C4/n0 : Integrator  InitialCondition=C0(4)
  C4/n0/tau_c(t) : Fcn  Expr=u[10]/(tau_c/u[2])
  C5/n0 : Integrator  InitialCondition=C0(5)
  C5/n0/tau_c(t) : Fcn  Expr=u[12]/(tau_c/u[2])
  C6/n0 : Integrator  InitialCondition=C0(6)
  C6/n0/tau_c(t) : Fcn  Expr=u[14]/(tau_c/u[2])
  Ci_delay1 : VariableTransportDelay  MaximumDelay=1000000  InitialOutput=C0(1)/tau_c
  Ci_delay2 : VariableTransportDelay  MaximumDelay=1000000  InitialOutput=C0(2)/tau_c
  Ci_delay3 : VariableTransportDelay  MaximumDelay=1000000  InitialOutput=C0(3)/tau_c
  Ci_delay4 : VariableTransportDelay  MaximumDelay=1000000  InitialOutput=C0(4)/tau_c
  Ci_delay5 : VariableTransportDelay  MaximumDelay=1000000  InitialOutput=C0(5)/tau_c
  Ci_delay6 : VariableTransportDelay  MaximumDelay=1000000  InitialOutput=C0(6)/tau_c
  Mux : Mux  Inputs=15
      settings: DisplayOption=signals
  Scope : Scope
  To Workspace : ToWorkspace  VariableName=core_pke  SampleTime=-1
  d(C1/n0)/dt : Fcn  Expr=(beta(1)*u[3]/Lam) - (lam(1)*u[4]) - (u[4]/(tau_c/u[2])) + (u[5]*exp(-lam(1)*tau_l/u[2]))
  d(C2/n0)/dt : Fcn  Expr=(beta(2)*u[3]/Lam) - (lam(2)*u[6]) - (u[6]/(tau_c/u[2])) + (u[7]*exp(-lam(2)*tau_l/u[2]))
  d(C3/n0)/dt : Fcn  Expr=(beta(3)*u[3]/Lam) - (lam(3)*u[8]) - (u[8]/(tau_c/u[2])) + (u[9]*exp(-lam(3)*tau_l/u[2]))
  d(C4/n0)/dt : Fcn  Expr=(beta(4)*u[3]/Lam) - (lam(4)*u[10]) - (u[10]/(tau_c/u[2])) + (u[11]*exp(-lam(4)*tau_l/u[2]))
  d(C5/n0)/dt : Fcn  Expr=(beta(5)*u[3]/Lam) - (lam(5)*u[12]) - (u[12]/(tau_c/u[2])) + (u[13]*exp(-lam(5)*tau_l/u[2]))
  d(C6/n0)/dt1 : Fcn  Expr=(beta(6)*u[3]/Lam) - (lam(6)*u[14]) - (u[14]/(tau_c/u[2])) + (u[14]*exp(-lam(6)*tau_l/u[2]))
  d(n/n0)/dt : Fcn  Expr=((u[1]-beta_t)*u[3]/Lam) + (lam(1)*u[4]) + (lam(2)*u[6]) + (lam(3)*u[8]) + (lam(4)*u[10]) + (lam(5)*u[12]) + (lam(6)*u[14])
  n/n0 : Integrator  InitialCondition=n0
  tau_l(t){1..6} (6 alike) : Fcn  Expr=tau_l/u[2]
  FRACTIONAL NEUTRON DENSITY : Outport
  wires:
  C1/n0/tau_c(t)/1 -> Ci_delay1/1
  d(n/n0)/dt/1 -> n/n0/1
  d(C1/n0)/dt/1 -> C1/n0/1
  REACTIVITY FEEDBACK/1 -> Mux/1
  n/n0/1 -> Scope/1, FRACTIONAL NEUTRON DENSITY/1, Mux/3
  FLOW FRACTION/1 -> Mux/2
  C1/n0/1 -> Mux/4
  Ci_delay1/1 -> Mux/5
  tau_l(t)1/1 -> Ci_delay1/2
  C2/n0/tau_c(t)/1 -> Ci_delay2/1
  d(C2/n0)/dt/1 -> C2/n0/1
  tau_l(t)2/1 -> Ci_delay2/2
  Ci_delay2/1 -> Mux/7
  C2/n0/1 -> Mux/6
  C3/n0/1 -> Mux/8
  d(C3/n0)/dt/1 -> C3/n0/1
  tau_l(t)3/1 -> Ci_delay3/2
  Ci_delay3/1 -> Mux/9
  C3/n0/tau_c(t)/1 -> Ci_delay3/1
  C4/n0/1 -> Mux/10
  C4/n0/tau_c(t)/1 -> Ci_delay4/1
  tau_l(t)4/1 -> Ci_delay4/2
  d(C4/n0)/dt/1 -> C4/n0/1
  Ci_delay4/1 -> Mux/11
  C5/n0/tau_c(t)/1 -> Ci_delay5/1
  d(C5/n0)/dt/1 -> C5/n0/1
  tau_l(t)5/1 -> Ci_delay5/2
  C5/n0/1 -> Mux/12
  Ci_delay5/1 -> Mux/13
  C6/n0/1 -> Mux/14
  tau_l(t)6/1 -> Ci_delay6/2
  d(C6/n0)/dt1/1 -> C6/n0/1
  C6/n0/tau_c(t)/1 -> Ci_delay6/1
  Ci_delay6/1 -> Mux/15
  Mux/1 -> To Workspace/1, tau_l(t)6/1, d(n/n0)/dt/1, d(C1/n0)/dt/1, C1/n0/tau_c(t)/1, tau_l(t)1/1, d(C2/n0)/dt/1, C2/n0/tau_c(t)/1, tau_l(t)2/1, d(C3/n0)/dt/1, C3/n0/tau_c(t)/1, tau_l(t)3/1, d(C4/n0)/dt/1, C4/n0/tau_c(t)/1, tau_l(t)4/1, d(C5/n0)/dt/1, C5/n0/tau_c(t)/1, tau_l(t)5/1, d(C6/n0)/dt1/1, C6/n0/tau_c(t)/1

== system MSDR_v1.1/CORE/REACTIVITY ==
  CORE TEMPERATURES : Inport
  XENON REACTIVITY : Inport  Port=2
  From Workspace : FromWorkspace  VariableName=react  SampleTime=1  Interpolate=off  OutputAfterFinalValue=Holding final value
  Sum1 : Sum
  Sum2 : Sum  Inputs=++++
  To Workspace : ToWorkspace  VariableName=core_react  SampleTime=-1
  dkf : Fcn  Expr=Ifa(1)*(u[3]-T0_fa(1)) + Ifb(1)*(u[4]-T0_fb(1)) + Ifa(2)*(u[6]-T0_fa(2)) + Ifb(2)*(u[7]-T0_fb(2))
  dkg : Fcn  Expr=Ig(1)*(u[5]-T0_g(1)) + Ig(2)*(u[8]-T0_g(2))
  fuel : Gain  Gain=a_f
  graphite : Gain  Gain=a_g
  rho_0 : Constant  Value=rho_0
  TOTAL REACTIVITY FEEDBACK : Outport
  wires:
  graphite/1 -> Sum1/2
  fuel/1 -> Sum1/1
  dkg/1 -> graphite/1
  dkf/1 -> fuel/1
  CORE TEMPERATURES/1 -> dkf/1, dkg/1
  Sum1/1 -> Sum2/2
  XENON REACTIVITY/1 -> Sum2/1
  Sum2/1 -> To Workspace/1, TOTAL REACTIVITY FEEDBACK/1
  rho_0/1 -> Sum2/3
  From Workspace/1 -> Sum2/4

== system MSDR_v1.1/CORE/REACTIVITY1 ==
  n0 : Inport
  Integrator1 : Integrator  InitialCondition=Xe_0
  Integrator2 : Integrator  InitialCondition=Xe_og
  Integrator30 : Integrator  InitialCondition=I_0
  Mux : Mux  Inputs=5
      settings: DisplayOption=signals
  Scope : Scope
  To Workspace : ToWorkspace  VariableName=msbr_poisons  SampleTime=-1
  Unit Delay : UnitDelay  SampleTime=-1
  d(I(t)/I0)/dt : Fcn  Expr=(gamma_I*Sig_f_msdr*phi_0)*u[1] - lam_I*u[2]
  d(Xe(t)/X0)/dt : Fcn  Expr=(gamma_Xe*Sig_f_msdr*phi_0)*u[1] + lam_I*u[2] - lam_Xe*u[3] - sig_Xe*phi_0*u[1]*u[3] - lam_bubl*u[3]
  d(Xe_og(t)/X0_og)/dt1 : Fcn  Expr=lam_bubl*u[3] - lam_Xe*u[4]
  drho_poison : Fcn  Expr=rhoXe_0*((u[3]/Xe_0)-1)
  drho_Xe : Outport
  wires:
  Integrator1/1 -> Scope/1, Mux/3
  Mux/1 -> d(Xe_og(t)/X0_og)/dt1/1, d(I(t)/I0)/dt/1, d(Xe(t)/X0)/dt/1, drho_poison/1, To Workspace/1
  Integrator2/1 -> Mux/4
  Unit Delay/1 -> Mux/5, drho_Xe/1
  n0/1 -> Mux/1
  drho_poison/1 -> Unit Delay/1
  d(Xe(t)/X0)/dt/1 -> Integrator1/1
  Integrator30/1 -> Mux/2
  d(Xe_og(t)/X0_og)/dt1/1 -> Integrator2/1
  d(I(t)/I0)/dt/1 -> Integrator30/1

== system MSDR_v1.1/HEAT EXCHANGERS/FUEL FLOW ==
  delay1 : Inport
  delay2 : Inport  Port=2
  delay3 : Inport  Port=3
  Fcn : Fcn  Expr=u[1]/3 + u[2]/3 + u[3]/3
  Mux : Mux
  Tf_out : Outport
  wires:
  delay1/1 -> Mux/1
  delay2/1 -> Mux/2
  delay3/1 -> Mux/3
  Fcn/1 -> Mux/4, Tf_out/1
  Mux/1 -> Fcn/1

== system MSDR_v1.1/HEAT EXCHANGERS/FUEL PUMP 1 ==
  1-D Lookup Table : Lookup_n-D  NumberOfTableDimensions=1  BreakpointsForDimension1=xdat  Table=ydat  InternalRulePriority=Speed  RndMeth=Simplest  InputSameDT=on
  Clock : Clock
  Fcn : Fcn  Expr=exp((1/tau_p)*u)
  Final convection flow rate : Constant  Value=therm_conv
  Scope : Scope
  Subtract : Sum  Inputs=-+
  Switch : Switch  Criteria=u2 > Threshold
  Transport Delay : TransportDelay  DelayTime=30000000  InitialOutput=1
  FLOW FRACTION : Outport
  HEAT TRANSFER FRACTION : Outport  Port=2
  wires:
  Transport Delay/1 -> 1-D Lookup Table/1, Scope/1, FLOW FRACTION/1
  Clock/1 -> Fcn/1
  Switch/1 -> Transport Delay/1
  Fcn/1 -> Subtract/1, Switch/1
  Final convection flow rate/1 -> Subtract/2, Switch/3
  Subtract/1 -> Switch/2
  1-D Lookup Table/1 -> HEAT TRANSFER FRACTION/1

== system MSDR_v1.1/HEAT EXCHANGERS/FUEL PUMP 2 ==
  1-D Lookup Table : Lookup_n-D  NumberOfTableDimensions=1  BreakpointsForDimension1=xdat  Table=ydat  InternalRulePriority=Speed  RndMeth=Simplest  InputSameDT=on
  Clock : Clock
  Fcn : Fcn  Expr=exp((1/tau_p)*u)
  Final convection flow rate : Constant  Value=therm_conv
  Scope : Scope
  Subtract : Sum  Inputs=-+
  Switch : Switch  Criteria=u2 > Threshold
  Transport Delay : TransportDelay  DelayTime=600000000  InitialOutput=1
  FLOW FRACTION : Outport
  HEAT TRANSFER FRACTION : Outport  Port=2
  wires:
  Transport Delay/1 -> 1-D Lookup Table/1, Scope/1, FLOW FRACTION/1
  Clock/1 -> Fcn/1
  Switch/1 -> Transport Delay/1
  Fcn/1 -> Subtract/1, Switch/1
  Final convection flow rate/1 -> Subtract/2, Switch/3
  Subtract/1 -> Switch/2
  1-D Lookup Table/1 -> HEAT TRANSFER FRACTION/1

== system MSDR_v1.1/HEAT EXCHANGERS/FUEL PUMP 3 ==
  1-D Lookup Table : Lookup_n-D  NumberOfTableDimensions=1  BreakpointsForDimension1=xdat  Table=ydat  InternalRulePriority=Speed  RndMeth=Simplest  InputSameDT=on
  Clock : Clock
  Fcn : Fcn  Expr=exp((1/tau_p)*u)
  Final convection flow rate : Constant  Value=therm_conv
  Scope : Scope
  Subtract : Sum  Inputs=-+
  Switch : Switch  Criteria=u2 > Threshold
  Transport Delay : TransportDelay  DelayTime=20000000  InitialOutput=1
  FLOW FRACTION : Outport
  HEAT TRANSFER FRACTION : Outport  Port=2
  wires:
  Transport Delay/1 -> 1-D Lookup Table/1, Scope/1, FLOW FRACTION/1
  Clock/1 -> Fcn/1
  Switch/1 -> Transport Delay/1
  Fcn/1 -> Subtract/1, Switch/1
  Final convection flow rate/1 -> Subtract/2, Switch/3
  Subtract/1 -> Switch/2
  1-D Lookup Table/1 -> HEAT TRANSFER FRACTION/1

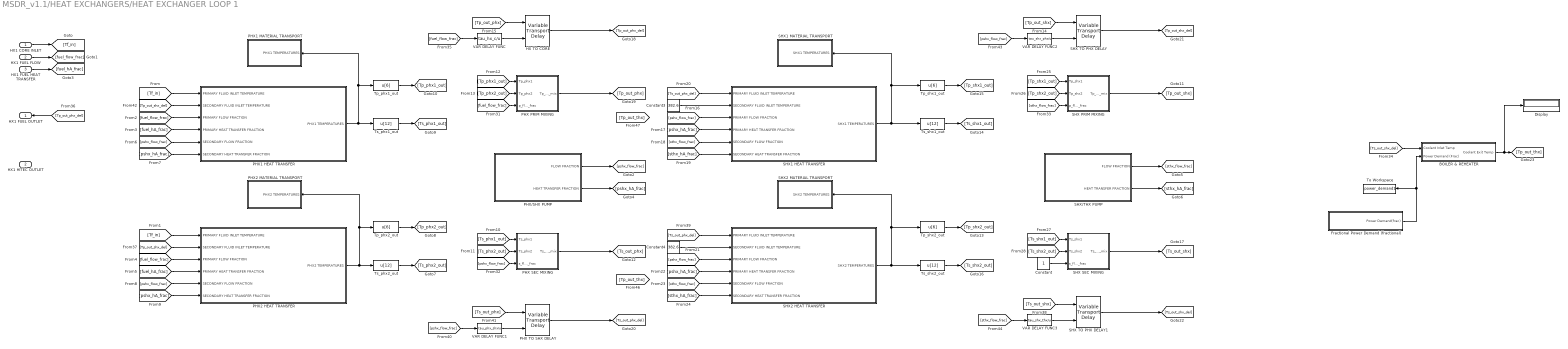
== system MSDR_v1.1/HEAT EXCHANGERS/HEAT EXCHANGER LOOP 1 ==
  HX1 CORE INLET : Inport
  HX1 FUEL FLOW : Inport  Port=2
  HX1 FUEL HEAT TRANSFER : Inport  Port=3
  BOILER & REHEATER : Subsystem
  Constant : Constant
  Constant3 : Constant  Value=382.6
  Constant4 : Constant  Value=382.6
  Display : Display
  Fractional Power Demand (fractional) : Subsystem
  HX TO CORE : VariableTransportDelay  MaximumDelay=1000000000000  InitialOutput=T0_p_phx1(4)
  PHX PRIM MIXING : Subsystem
  PHX SEC MIXING : Subsystem
  PHX TO SHX DELAY : VariableTransportDelay  MaximumDelay=100000000000  InitialOutput=T0_s_phx1(4)
  PHX/SHX PUMP : Subsystem
  PHX1 HEAT TRANSFER : Subsystem
  PHX1 MATERIAL TRANSPORT : Subsystem
  PHX2 HEAT TRANSFER : Subsystem
  PHX2 MATERIAL TRANSPORT : Subsystem
  SHX PRIM MIXING : Subsystem
  SHX SEC MIXING : Subsystem
  SHX TO PHX DELAY : VariableTransportDelay  MaximumDelay=1000000000000  InitialOutput=T0_p_shx1(4)
  SHX TO PHX DELAY1 : VariableTransportDelay  MaximumDelay=1000000000000  InitialOutput=T0_s_shx1(4)
  SHX/THX PUMP : Subsystem
  SHX1 HEAT TRANSFER : Subsystem
  SHX1 MATERIAL TRANSPORT : Subsystem
  SHX2 HEAT TRANSFER : Subsystem
  SHX2 MATERIAL TRANSPORT : Subsystem
  To Workspace : ToWorkspace  VariableName=power_demand1  SampleTime=-1
  Tp_phx1_out : Fcn  Expr=u[6]
  Tp_phx2_out : Fcn  Expr=u[6]
  Tp_shx1_out : Fcn  Expr=u[6]
  Tp_shx2_out : Fcn  Expr=u[6]
  Ts_phx1_out : Fcn  Expr=u[12]
  Ts_phx2_out : Fcn  Expr=u[12]
  Ts_shx1_out : Fcn  Expr=u[12]
  Ts_shx2_out : Fcn  Expr=u[12]
  VAR DELAY FUNC : Fcn  Expr=tau_hx_c/u
  VAR DELAY FUNC1 : Fcn  Expr=tau_phx_shx/u
  VAR DELAY FUNC2 : Fcn  Expr=tau_shx_phx/u
  VAR DELAY FUNC3 : Fcn  Expr=tau_shx_thx/u
  HX1 FUEL OUTLET : Outport
  HX1 HITEC OUTLET : Outport  Port=2
  wires:
  PHX1 HEAT TRANSFER/1(PHX1 TEMPERATURES) -> PHX1 MATERIAL TRANSPORT/1(PHX1 TEMPERATURES), Tp_phx1_out/1, Ts_phx1_out/1
  SHX1 HEAT TRANSFER/1(SHX1 TEMPERATURES) -> Ts_shx1_out/1, Tp_shx1_out/1, SHX1 MATERIAL TRANSPORT/1(SHX1 TEMPERATURES)
  PHX2 HEAT TRANSFER/1(PHX2 TEMPERATURES) -> PHX2 MATERIAL TRANSPORT/1(PHX2 TEMPERATURES), Tp_phx2_out/1, Ts_phx2_out/1
  SHX2 HEAT TRANSFER/1(SHX2 TEMPERATURES) -> Ts_shx2_out/1, SHX2 MATERIAL TRANSPORT/1(SHX2 TEMPERATURES), Tp_shx2_out/1
  HX1 CORE INLET/1 -> [Tf_in]
  [Tf_in] -> PHX1 HEAT TRANSFER/1(PRIMARY FLUID INLET TEMPERATURE)
  [Tf_in] -> PHX2 HEAT TRANSFER/1(PRIMARY FLUID INLET TEMPERATURE)
  HX1 FUEL FLOW/1 -> [fuel_flow_frac]
  HX1 FUEL HEAT TRANSFER/1 -> [fuel_hA_frac]
  [fuel_flow_frac] -> PHX1 HEAT TRANSFER/3(PRIMARY FLOW FRACTION)
  [fuel_hA_frac] -> PHX1 HEAT TRANSFER/4(PRIMARY HEAT TRANSFER FRACTION)
  [fuel_flow_frac] -> PHX2 HEAT TRANSFER/3(PRIMARY FLOW FRACTION)
  [fuel_hA_frac] -> PHX2 HEAT TRANSFER/4(PRIMARY HEAT TRANSFER FRACTION)
  PHX/SHX PUMP/2(HEAT TRANSFER FRACTION) -> [pshx_hA_frac]
  PHX/SHX PUMP/1(FLOW FRACTION) -> [pshx_flow_frac]
  SHX/THX PUMP/1(FLOW FRACTION) -> [sthx_flow_frac]
  SHX/THX PUMP/2(HEAT TRANSFER FRACTION) -> [sthx_hA_frac]
  Ts_phx2_out/1 -> [Ts_phx2_out]
  Tp_phx2_out/1 -> [Tp_phx2_out]
  Tp_phx1_out/1 -> [Tp_phx1_out]
  Ts_phx1_out/1 -> [Ts_phx1_out]
  [pshx_flow_frac] -> PHX1 HEAT TRANSFER/5(SECONDARY FLOW FRACTION)
  [pshx_hA_frac] -> PHX1 HEAT TRANSFER/6(SECONDARY HEAT TRANSFER FRACTION)
  [pshx_flow_frac] -> PHX2 HEAT TRANSFER/5(SECONDARY FLOW FRACTION)
  [pshx_hA_frac] -> PHX2 HEAT TRANSFER/6(SECONDARY HEAT TRANSFER FRACTION)
  [Tp_phx1_out] -> PHX PRIM MIXING/1(Tp_phx1)
  [Tp_phx2_out] -> PHX PRIM MIXING/2(Tp_phx2)
  PHX PRIM MIXING/1(Tp_phx_mix) -> [Tp_out_phx]
  [Ts_out_phx_del] -> SHX1 HEAT TRANSFER/1(PRIMARY FLUID INLET TEMPERATURE)
  [pshx_flow_frac] -> SHX1 HEAT TRANSFER/3(PRIMARY FLOW FRACTION)
  [pshx_hA_frac] -> SHX1 HEAT TRANSFER/4(PRIMARY HEAT TRANSFER FRACTION)
  [sthx_flow_frac] -> SHX1 HEAT TRANSFER/5(SECONDARY FLOW FRACTION)
  [sthx_hA_frac] -> SHX1 HEAT TRANSFER/6(SECONDARY HEAT TRANSFER FRACTION)
  [Ts_out_phx_del] -> SHX2 HEAT TRANSFER/1(PRIMARY FLUID INLET TEMPERATURE)
  [pshx_flow_frac] -> SHX2 HEAT TRANSFER/3(PRIMARY FLOW FRACTION)
  [pshx_hA_frac] -> SHX2 HEAT TRANSFER/4(PRIMARY HEAT TRANSFER FRACTION)
  [sthx_flow_frac] -> SHX2 HEAT TRANSFER/5(SECONDARY FLOW FRACTION)
  [sthx_hA_frac] -> SHX2 HEAT TRANSFER/6(SECONDARY HEAT TRANSFER FRACTION)
  Tp_shx1_out/1 -> [Tp_shx1_out]
  Tp_shx2_out/1 -> [Tp_shx2_out]
  Ts_shx1_out/1 -> [Ts_shx1_out]
  Ts_shx2_out/1 -> [Ts_shx2_out]
  [fuel_flow_frac] -> PHX PRIM MIXING/3(p_flow_frac)
  [pshx_flow_frac] -> PHX SEC MIXING/3(s_flow_frac)
  [Ts_phx2_out] -> PHX SEC MIXING/2(Ts_phx2)
  [Ts_phx1_out] -> PHX SEC MIXING/1(Ts_phx1)
  PHX SEC MIXING/1(Ts_phx_mix) -> [Ts_out_phx]
  [sthx_flow_frac] -> SHX PRIM MIXING/3(p_flow_frac)
  [Tp_shx2_out] -> SHX PRIM MIXING/2(Tp_shx2)
  [Tp_shx1_out] -> SHX PRIM MIXING/1(Tp_shx1)
  SHX PRIM MIXING/1(Tp_shx_mix) -> [Tp_out_shx]
  [Ts_shx1_out] -> SHX SEC MIXING/1(Ts_shx1)
  SHX SEC MIXING/1(Ts_shx_mix) -> [Ts_out_shx]
  [Ts_shx2_out] -> SHX SEC MIXING/2(Ts_shx2)
  Constant/1 -> SHX SEC MIXING/3(s_flow_frac)
  [Tp_out_shx_del] -> PHX1 HEAT TRANSFER/2(SECONDARY FLUID INLET TEMPERATURE)
  [Tp_out_shx_del] -> PHX2 HEAT TRANSFER/2(SECONDARY FLUID INLET TEMPERATURE)
  VAR DELAY FUNC/1 -> HX TO CORE/2
  [Tp_out_phx] -> HX TO CORE/1
  [fuel_flow_frac] -> VAR DELAY FUNC/1
  HX TO CORE/1 -> [Tp_out_phx_del]
  [Tp_out_phx_del] -> HX1 FUEL OUTLET/1
  VAR DELAY FUNC1/1 -> PHX TO SHX DELAY/2
  PHX TO SHX DELAY/1 -> [Ts_out_phx_del]
  [Ts_out_phx] -> PHX TO SHX DELAY/1
  [pshx_flow_frac] -> VAR DELAY FUNC1/1
  VAR DELAY FUNC2/1 -> SHX TO PHX DELAY/2
  SHX TO PHX DELAY/1 -> [Tp_out_shx_del]
  [pshx_flow_frac] -> VAR DELAY FUNC2/1
  [Tp_out_shx] -> SHX TO PHX DELAY/1
  [Ts_out_shx] -> SHX TO PHX DELAY1/1
  [sthx_flow_frac] -> VAR DELAY FUNC3/1
  SHX TO PHX DELAY1/1 -> [Ts_out_shx_del]
  VAR DELAY FUNC3/1 -> SHX TO PHX DELAY1/2
  Fractional Power Demand (fractional)/1(Power Demand(frac)) -> BOILER & REHEATER/2(Power Demand (Frac)), To Workspace/1
  [Ts_out_shx_del] -> BOILER & REHEATER/1(Coolant Inlet Temp)
  BOILER & REHEATER/1(Coolant Exit Temp) -> Display/1, [Tp_out_thx]
  Constant3/1 -> SHX1 HEAT TRANSFER/2(SECONDARY FLUID INLET TEMPERATURE)
  Constant4/1 -> SHX2 HEAT TRANSFER/2(SECONDARY FLUID INLET TEMPERATURE)

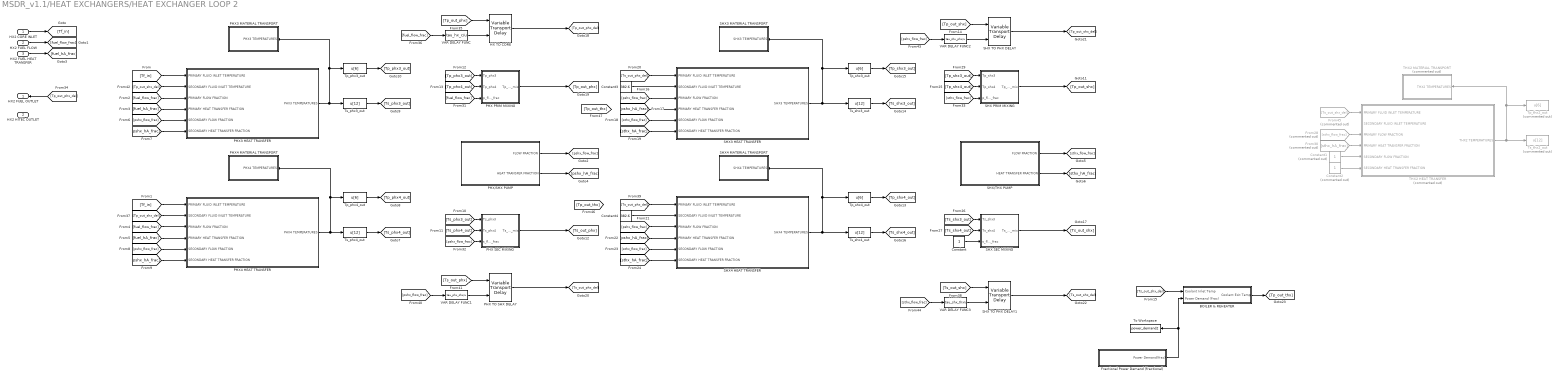
== system MSDR_v1.1/HEAT EXCHANGERS/HEAT EXCHANGER LOOP 2 ==
  HX2 CORE INLET : Inport
  HX2 FUEL FLOW : Inport  Port=2
  HX2 FUEL HEAT TRANSFER : Inport  Port=3
  BOILER & REHEATER : Subsystem
  Constant : Constant
  Constant1 : Constant  Commented=on
  Constant2 : Constant  Commented=on
  Constant3 : Constant  Value=382.6
  Constant4 : Constant  Value=382.6
  Fractional Power Demand (fractional) : Subsystem
  From28 : From  Commented=on  GotoTag=sthx_flow_frac
  From30 : From  Commented=on  GotoTag=sthx_hA_frac
  From45 : From  Commented=on  GotoTag=Ts_out_shx_del
  HX TO CORE : VariableTransportDelay  MaximumDelay=1000000000000  InitialOutput=T0_p_phx3(4)
  PHX PRIM MIXING : Subsystem
  PHX SEC MIXING : Subsystem
  PHX TO SHX DELAY : VariableTransportDelay  MaximumDelay=100000000000  InitialOutput=T0_s_phx3(4)
  PHX/SHX PUMP : Subsystem
  PHX3 HEAT TRANSFER : Subsystem
  PHX3 MATERIAL TRANSPORT : Subsystem
  PHX4 HEAT TRANSFER : Subsystem
  PHX4 MATERIAL TRANSPORT : Subsystem
  SHX PRIM MIXING : Subsystem
  SHX SEC MIXING : Subsystem
  SHX TO PHX DELAY : VariableTransportDelay  MaximumDelay=1000000000000  InitialOutput=T0_p_shx3(4)
  SHX TO PHX DELAY1 : VariableTransportDelay  MaximumDelay=1000000000000  InitialOutput=T0_s_shx3(4)
  SHX/THX PUMP : Subsystem
  SHX3 HEAT TRANSFER : Subsystem
  SHX3 MATERIAL TRANSPORT : Subsystem
  SHX4 HEAT TRANSFER : Subsystem
  SHX4 MATERIAL TRANSPORT : Subsystem
  THX2 HEAT TRANSFER : Subsystem  Commented=on
  THX2 MATERIAL TRANSPORT : Subsystem  Commented=on
  To Workspace : ToWorkspace  VariableName=power_demand2  SampleTime=-1
  Tp_phx3_out : Fcn  Expr=u[6]
  Tp_phx4_out : Fcn  Expr=u[6]
  Tp_shx3_out : Fcn  Expr=u[6]
  Tp_shx4_out : Fcn  Expr=u[6]
  Tp_thx2_out : Fcn  Commented=on  Expr=u[6]
  Ts_phx3_out : Fcn  Expr=u[12]
  Ts_phx4_out : Fcn  Expr=u[12]
  Ts_shx3_out : Fcn  Expr=u[12]
  Ts_shx4_out : Fcn  Expr=u[12]
  Ts_thx2_out : Fcn  Commented=on  Expr=u[12]
  VAR DELAY FUNC : Fcn  Expr=tau_hx_c/u
  VAR DELAY FUNC1 : Fcn  Expr=tau_phx_shx/u
  VAR DELAY FUNC2 : Fcn  Expr=tau_shx_phx/u
  VAR DELAY FUNC3 : Fcn  Expr=tau_shx_thx/u
  HX2 FUEL OUTLET : Outport
  HX2 HITEC OUTLET : Outport  Port=2
  wires:
  [Tp_out_phx_del] -> HX2 FUEL OUTLET/1
  HX2 CORE INLET/1 -> [Tf_in]
  HX2 FUEL HEAT TRANSFER/1 -> [fuel_hA_frac]
  HX2 FUEL FLOW/1 -> [fuel_flow_frac]
  Tp_phx3_out/1 -> [Tp_phx3_out]
  PHX3 HEAT TRANSFER/1(PHX3 TEMPERATURES) -> PHX3 MATERIAL TRANSPORT/1(PHX3 TEMPERATURES), Tp_phx3_out/1, Ts_phx3_out/1
  Ts_phx3_out/1 -> [Ts_phx3_out]
  Tp_phx4_out/1 -> [Tp_phx4_out]
  Ts_phx4_out/1 -> [Ts_phx4_out]
  PHX4 HEAT TRANSFER/1(PHX4 TEMPERATURES) -> PHX4 MATERIAL TRANSPORT/1(PHX4 TEMPERATURES), Tp_phx4_out/1, Ts_phx4_out/1
  Tp_shx3_out/1 -> [Tp_shx3_out]
  Ts_shx3_out/1 -> [Ts_shx3_out]
  SHX3 HEAT TRANSFER/1(SHX3 TEMPERATURES) -> Ts_shx3_out/1, SHX3 MATERIAL TRANSPORT/1(SHX3 TEMPERATURES), Tp_shx3_out/1
  [Tp_phx3_out] -> PHX PRIM MIXING/1(Tp_phx3)
  [fuel_flow_frac] -> PHX PRIM MIXING/3(p_flow_frac)
  [Ts_phx3_out] -> PHX SEC MIXING/1(Ts_phx3)
  [Ts_phx4_out] -> PHX SEC MIXING/2(Ts_phx4)
  [Tp_phx4_out] -> PHX PRIM MIXING/2(Tp_phx4)
  PHX SEC MIXING/1(Ts_phx_mix) -> [Ts_out_phx]
  PHX/SHX PUMP/1(FLOW FRACTION) -> [pshx_flow_frac]
  PHX PRIM MIXING/1(Tp_phx_mix) -> [Tp_out_phx]
  [pshx_flow_frac] -> PHX SEC MIXING/3(s_flow_frac)
  PHX/SHX PUMP/2(HEAT TRANSFER FRACTION) -> [pshx_hA_frac]
  Tp_shx4_out/1 -> [Tp_shx4_out]
  SHX4 HEAT TRANSFER/1(SHX4 TEMPERATURES) -> Ts_shx4_out/1, SHX4 MATERIAL TRANSPORT/1(SHX4 TEMPERATURES), Tp_shx4_out/1
  Ts_shx4_out/1 -> [Ts_shx4_out]
  [Tp_shx3_out] -> SHX PRIM MIXING/1(Tp_shx3)
  [Ts_shx4_out] -> SHX SEC MIXING/2(Ts_shx4)
  [Ts_shx3_out] -> SHX SEC MIXING/1(Ts_shx3)
  [Tp_shx4_out] -> SHX PRIM MIXING/2(Tp_shx4)
  SHX/THX PUMP/2(HEAT TRANSFER FRACTION) -> [sthx_hA_frac]
  SHX SEC MIXING/1(Ts_shx_mix) -> [Ts_out_shx]
  SHX PRIM MIXING/1(Tp_shx_mix) -> [Tp_out_shx]
  SHX/THX PUMP/1(FLOW FRACTION) -> [sthx_flow_frac]
  [sthx_flow_frac] -> SHX PRIM MIXING/3(p_flow_frac)
  Constant/1 -> SHX SEC MIXING/3(s_flow_frac)
  THX2 HEAT TRANSFER/1(THX2 TEMPERATURES) -> THX2 MATERIAL TRANSPORT/1(THX2 TEMPERATURES), Tp_thx2_out/1, Ts_thx2_out/1
  [fuel_hA_frac] -> PHX3 HEAT TRANSFER/4(PRIMARY HEAT TRANSFER FRACTION)
  [Tp_out_shx_del] -> PHX3 HEAT TRANSFER/2(SECONDARY FLUID INLET TEMPERATURE)
  [pshx_hA_frac] -> PHX3 HEAT TRANSFER/6(SECONDARY HEAT TRANSFER FRACTION)
  [Tf_in] -> PHX3 HEAT TRANSFER/1(PRIMARY FLUID INLET TEMPERATURE)
  [pshx_flow_frac] -> PHX3 HEAT TRANSFER/5(SECONDARY FLOW FRACTION)
  [fuel_flow_frac] -> PHX3 HEAT TRANSFER/3(PRIMARY FLOW FRACTION)
  [Tp_out_shx_del] -> PHX4 HEAT TRANSFER/2(SECONDARY FLUID INLET TEMPERATURE)
  [pshx_flow_frac] -> PHX4 HEAT TRANSFER/5(SECONDARY FLOW FRACTION)
  [fuel_flow_frac] -> PHX4 HEAT TRANSFER/3(PRIMARY FLOW FRACTION)
  [Tf_in] -> PHX4 HEAT TRANSFER/1(PRIMARY FLUID INLET TEMPERATURE)
  [pshx_hA_frac] -> PHX4 HEAT TRANSFER/6(SECONDARY HEAT TRANSFER FRACTION)
  [fuel_hA_frac] -> PHX4 HEAT TRANSFER/4(PRIMARY HEAT TRANSFER FRACTION)
  VAR DELAY FUNC/1 -> HX TO CORE/2
  HX TO CORE/1 -> [Tp_out_phx_del]
  [Tp_out_phx] -> HX TO CORE/1
  [fuel_flow_frac] -> VAR DELAY FUNC/1
  [Ts_out_phx] -> PHX TO SHX DELAY/1
  [pshx_flow_frac] -> VAR DELAY FUNC1/1
  VAR DELAY FUNC1/1 -> PHX TO SHX DELAY/2
  PHX TO SHX DELAY/1 -> [Ts_out_phx_del]
  [sthx_flow_frac] -> SHX3 HEAT TRANSFER/5(SECONDARY FLOW FRACTION)
  [sthx_hA_frac] -> SHX3 HEAT TRANSFER/6(SECONDARY HEAT TRANSFER FRACTION)
  [pshx_hA_frac] -> SHX3 HEAT TRANSFER/4(PRIMARY HEAT TRANSFER FRACTION)
  [Ts_out_phx_del] -> SHX3 HEAT TRANSFER/1(PRIMARY FLUID INLET TEMPERATURE)
  [pshx_flow_frac] -> SHX3 HEAT TRANSFER/3(PRIMARY FLOW FRACTION)
  [sthx_hA_frac] -> SHX4 HEAT TRANSFER/6(SECONDARY HEAT TRANSFER FRACTION)
  [sthx_flow_frac] -> SHX4 HEAT TRANSFER/5(SECONDARY FLOW FRACTION)
  [pshx_hA_frac] -> SHX4 HEAT TRANSFER/4(PRIMARY HEAT TRANSFER FRACTION)
  [pshx_flow_frac] -> SHX4 HEAT TRANSFER/3(PRIMARY FLOW FRACTION)
  [Ts_out_phx_del] -> SHX4 HEAT TRANSFER/1(PRIMARY FLUID INLET TEMPERATURE)
  [Tp_out_shx] -> SHX TO PHX DELAY/1
  [pshx_flow_frac] -> VAR DELAY FUNC2/1
  SHX TO PHX DELAY/1 -> [Tp_out_shx_del]
  VAR DELAY FUNC2/1 -> SHX TO PHX DELAY/2
  VAR DELAY FUNC3/1 -> SHX TO PHX DELAY1/2
  SHX TO PHX DELAY1/1 -> [Ts_out_shx_del]
  [Ts_out_shx] -> SHX TO PHX DELAY1/1
  [sthx_flow_frac] -> VAR DELAY FUNC3/1
  From30/1 -> THX2 HEAT TRANSFER/4(PRIMARY HEAT TRANSFER FRACTION)
  From45/1 -> THX2 HEAT TRANSFER/1(PRIMARY FLUID INLET TEMPERATURE)
  Constant1/1 -> THX2 HEAT TRANSFER/5(SECONDARY FLOW FRACTION)
  Constant2/1 -> THX2 HEAT TRANSFER/6(SECONDARY HEAT TRANSFER FRACTION)
  From28/1 -> THX2 HEAT TRANSFER/3(PRIMARY FLOW FRACTION)
  BOILER & REHEATER/1(Coolant Exit Temp) -> [Tp_out_thx]
  [Ts_out_shx_del] -> BOILER & REHEATER/1(Coolant Inlet Temp)
  Fractional Power Demand (fractional)/1(Power Demand(frac)) -> BOILER & REHEATER/2(Power Demand (Frac)), To Workspace/1
  Constant3/1 -> SHX3 HEAT TRANSFER/2(SECONDARY FLUID INLET TEMPERATURE)
  Constant4/1 -> SHX4 HEAT TRANSFER/2(SECONDARY FLUID INLET TEMPERATURE)
